simulink model "lab_4s"  (R2016a)
settings: Solver=VariableStepAuto  StartTime=0.0  StopTime=10.0  RelTol=1e-3
libraries: simulink x2
settings Model: Creator=Anthunder  LastModifiedBy=Anthunder

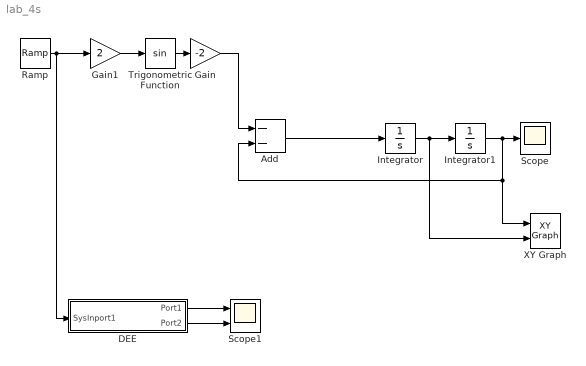
== system lab_4s ==
  Add : Sum  Inputs=--
  DEE : Subsystem  mask(Differential Equation Editor (DEE)){}
      settings: OpenFcn=diffeqed
      mask Display: disp('Differential Equation\n Editor')
  Gain : Gain  Gain=-2
  Gain1 : Gain  Gain=2
  Integrator : Integrator
  Integrator1 : Integrator
  Ramp : simulink/Sources/Ramp  slope=1  start=0  X0=0
  Scope : Scope
  Scope1 : Scope  NumInputPorts=2
  Trigonometric Function : Trigonometry
  XY Graph : simulink/Sinks/XY Graph  xmin=-1  xmax=1  ymin=-1  ymax=1  st=-1
  wires:
  Ramp/1 -> Gain1/1, DEE/1(SysInport1)
  Trigonometric Function/1 -> Gain/1
  Integrator/1 -> XY Graph/2, Integrator1/1
  Add/1 -> Integrator/1
  Integrator1/1 -> Add/2, XY Graph/1, Scope/1
  Gain/1 -> Add/1
  DEE/1(Port1) -> Scope1/1
  DEE/2(Port2) -> Scope1/2
  Gain1/1 -> Trigonometric Function/1

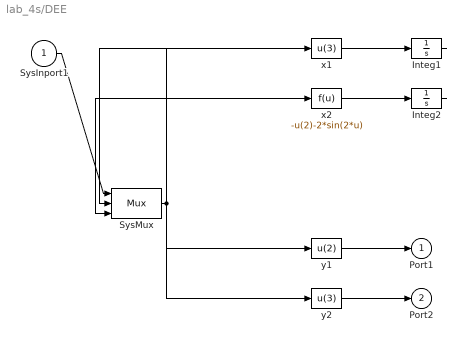
== system lab_4s/DEE ==
  SysInport1 : Inport
  Integ1 : Integrator  InitialCondition=1
  Integ2 : Integrator  InitialCondition=1
  SysMux : Mux  Inputs=3
  x1 : Fcn  Expr=u(3)
  x2 : Fcn  Expr=-u(2)-2*sin(2*u)
  y1 : Fcn  Expr=u(2)
  y2 : Fcn  Expr=u(3)
  Port1 : Outport
  Port2 : Outport  Port=2
  wires:
  SysInport1/1 -> SysMux/1
  SysMux/1 -> x1/1, x2/1, y1/1, y2/1
  x1/1 -> Integ1/1
  Integ1/1 -> SysMux/2
  x2/1 -> Integ2/1
  Integ2/1 -> SysMux/3
  y1/1 -> Port1/1
  y2/1 -> Port2/1
